simulink model "CC3"  (Simulink 7.5)
settings: Solver=ode45  StartTime=0.0  StopTime=2  RelTol=1e-3
(part 1 of 2)
settings Model: Creator=Fer  LastModifiedBy=Fer

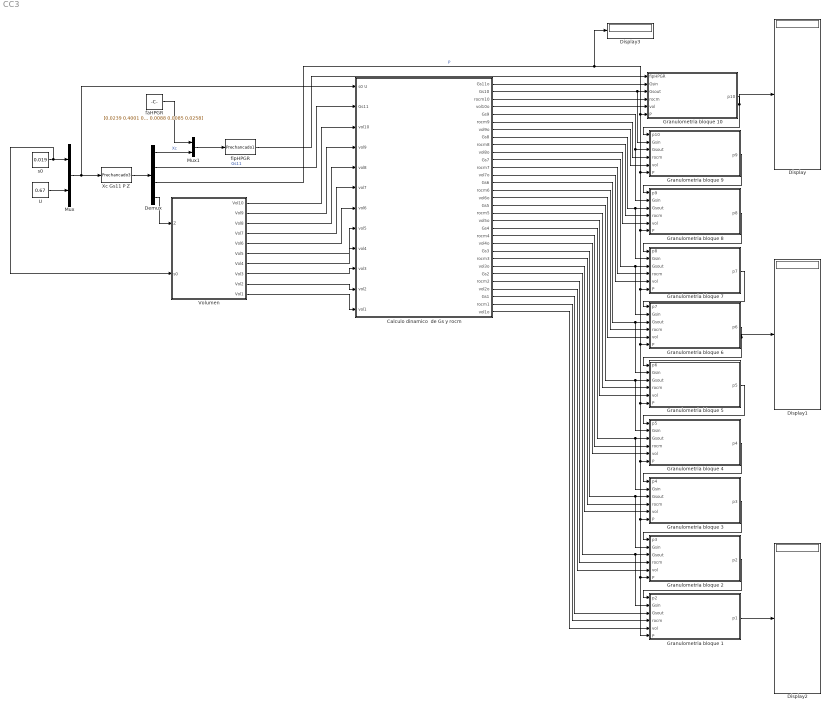
== system CC3 ==
  Calculo dinamico  de Gs y rocm : Subsystem
  Demux : Demux
  Display{,1..3} (4 alike) : Display
  Granulometria bloque 1 : Subsystem
  Granulometria bloque 10 : Subsystem
  Granulometria bloque 2 : Subsystem
  Granulometria bloque 3 : Subsystem
  Granulometria bloque 4 : Subsystem
  Granulometria bloque 5 : Subsystem
  Granulometria bloque 6 : Subsystem
  Granulometria bloque 7 : Subsystem
  Granulometria bloque 8 : Subsystem
  Granulometria bloque 9 : Subsystem
  Mux : Mux  Inputs=2
  Mux1 : Mux  Inputs=2
  U : Constant  Value=0.67  OutDataType=fixdt(1, 16)  OutScaling=2^0
  Volumen : Subsystem
  Xc Gs11 P Z : MATLABFcn  MATLABFcn=Prechancado3
  faHPGR : Constant  Value=[0.0239 0.4001 0.2089 0.1090 0.0549 0.0441 0.0542 0.0374 0.0159 0.0085 0.0088 0.0085 0.0258]  OutDataType=fixdt(1, 16)  OutScaling=2^0
  fipHPGR : MATLABFcn  MATLABFcn=Prechancado1
  s0 : Constant  Value=0.019  OutDataType=fixdt(1, 16)  OutScaling=2^0
  wires:
  s0/1 -> Mux/1, Volumen/2(s0)
  U/1 -> Mux/2
  Mux/1 -> Xc Gs11 P Z/1, Calculo dinamico  de Gs y rocm/1(s0 U)
  Xc Gs11 P Z/1 -> Demux/1
  faHPGR/1 -> Mux1/1
  Demux/1 -> Mux1/2  "Xc"
  Mux1/1 -> fipHPGR/1
  Demux/2 -> Calculo dinamico  de Gs y rocm/2(Gs11)  "Gs11"
  Volumen/1(Vol10) -> Calculo dinamico  de Gs y rocm/3(vol10)
  Volumen/2(Vol9) -> Calculo dinamico  de Gs y rocm/4(vol9)
  Volumen/3(Vol8) -> Calculo dinamico  de Gs y rocm/5(vol8)
  Volumen/4(Vol7) -> Calculo dinamico  de Gs y rocm/6(vol7)
  Volumen/5(Vol6) -> Calculo dinamico  de Gs y rocm/7(vol6)
  Volumen/6(Vol5) -> Calculo dinamico  de Gs y rocm/8(vol5)
  Volumen/7(Vol4) -> Calculo dinamico  de Gs y rocm/9(vol4)
  Volumen/8(Vol3) -> Calculo dinamico  de Gs y rocm/10(vol3)
  Volumen/9(Vol2) -> Calculo dinamico  de Gs y rocm/11(vol2)
  Volumen/10(Vol1) -> Calculo dinamico  de Gs y rocm/12(vol1)
  fipHPGR/1 -> Granulometria bloque 10/1(fipHPGR)
  Calculo dinamico  de Gs y rocm/1(Gs11o) -> Granulometria bloque 10/2(Gsin)
  Calculo dinamico  de Gs y rocm/2(Gs10) -> Granulometria bloque 10/3(Gsout), Granulometria bloque 9/2(Gsin)
  Calculo dinamico  de Gs y rocm/3(rocm10) -> Granulometria bloque 10/4(rocm)
  Calculo dinamico  de Gs y rocm/4(vol10o) -> Granulometria bloque 10/5(vol)
  Demux/4 -> Volumen/1(Z)
  Demux/3 -> Granulometria bloque 10/6(P), Granulometria bloque 9/6(P), Granulometria bloque 8/6(P), Granulometria bloque 7/6(P), Granulometria bloque 6/6(P), Granulometria bloque 5/6(P), Granulometria bloque 4/6(P), Granulometria bloque 3/6(P), Granulometria bloque 2/6(P), Granulometria bloque 1/6(P), Display3/1  "P"
  Granulometria bloque 10/1(p10) -> Granulometria bloque 9/1(p10), Display/1
  Calculo dinamico  de Gs y rocm/5(Gs9) -> Granulometria bloque 9/3(Gsout), Granulometria bloque 8/2(Gsin)
  Calculo dinamico  de Gs y rocm/6(rocm9) -> Granulometria bloque 9/4(rocm)
  Calculo dinamico  de Gs y rocm/7(vol9o) -> Granulometria bloque 9/5(vol)
  Granulometria bloque 9/1(p9) -> Granulometria bloque 8/1(p9)
  Calculo dinamico  de Gs y rocm/8(Gs8) -> Granulometria bloque 8/3(Gsout), Granulometria bloque 7/2(Gsin)
  Calculo dinamico  de Gs y rocm/9(rocm8) -> Granulometria bloque 8/4(rocm)
  Calculo dinamico  de Gs y rocm/10(vol8o) -> Granulometria bloque 8/5(vol)
  Granulometria bloque 8/1(p8) -> Granulometria bloque 7/1(p8)
  Calculo dinamico  de Gs y rocm/11(Gs7) -> Granulometria bloque 7/3(Gsout), Granulometria bloque 6/2(Gsin)
  Calculo dinamico  de Gs y rocm/12(rocm7) -> Granulometria bloque 7/4(rocm)
  Calculo dinamico  de Gs y rocm/13(vol7o) -> Granulometria bloque 7/5(vol)
  Granulometria bloque 7/1(p7) -> Granulometria bloque 6/1(p7)
  Calculo dinamico  de Gs y rocm/14(Gs6) -> Granulometria bloque 6/3(Gsout), Granulometria bloque 5/2(Gsin)
  Calculo dinamico  de Gs y rocm/15(rocm6) -> Granulometria bloque 6/4(rocm)
  Calculo dinamico  de Gs y rocm/16(vol6o) -> Granulometria bloque 6/5(vol)
  Granulometria bloque 6/1(p6) -> Granulometria bloque 5/1(p6), Display1/1
  Calculo dinamico  de Gs y rocm/17(Gs5) -> Granulometria bloque 5/3(Gsout), Granulometria bloque 4/2(Gsin)
  Calculo dinamico  de Gs y rocm/18(rocm5) -> Granulometria bloque 5/4(rocm)
  Calculo dinamico  de Gs y rocm/19(vol5o) -> Granulometria bloque 5/5(vol)
  Granulometria bloque 5/1(p5) -> Granulometria bloque 4/1(p5)
  Calculo dinamico  de Gs y rocm/20(Gs4) -> Granulometria bloque 4/3(Gsout), Granulometria bloque 3/2(Gsin)
  Calculo dinamico  de Gs y rocm/21(rocm4) -> Granulometria bloque 4/4(rocm)
  Calculo dinamico  de Gs y rocm/22(vol4o) -> Granulometria bloque 4/5(vol)
  Granulometria bloque 4/1(p4) -> Granulometria bloque 3/1(p4)
  Calculo dinamico  de Gs y rocm/23(Gs3) -> Granulometria bloque 3/3(Gsout), Granulometria bloque 2/2(Gsin)
  Calculo dinamico  de Gs y rocm/24(rocm3) -> Granulometria bloque 3/4(rocm)
  Calculo dinamico  de Gs y rocm/25(vol3o) -> Granulometria bloque 3/5(vol)
  Granulometria bloque 3/1(p3) -> Granulometria bloque 2/1(p3)
  Calculo dinamico  de Gs y rocm/26(Gs2) -> Granulometria bloque 2/3(Gsout), Granulometria bloque 1/2(Gsin)
  Calculo dinamico  de Gs y rocm/27(rocm2) -> Granulometria bloque 2/4(rocm)
  Calculo dinamico  de Gs y rocm/28(vol2o) -> Granulometria bloque 2/5(vol)
  Granulometria bloque 2/1(p2) -> Granulometria bloque 1/1(p2)
  Calculo dinamico  de Gs y rocm/29(Gs1) -> Granulometria bloque 1/3(Gsout)
  Calculo dinamico  de Gs y rocm/30(rocm1) -> Granulometria bloque 1/4(rocm)
  Calculo dinamico  de Gs y rocm/31(vol1o) -> Granulometria bloque 1/5(vol)
  Granulometria bloque 1/1(p1) -> Display2/1

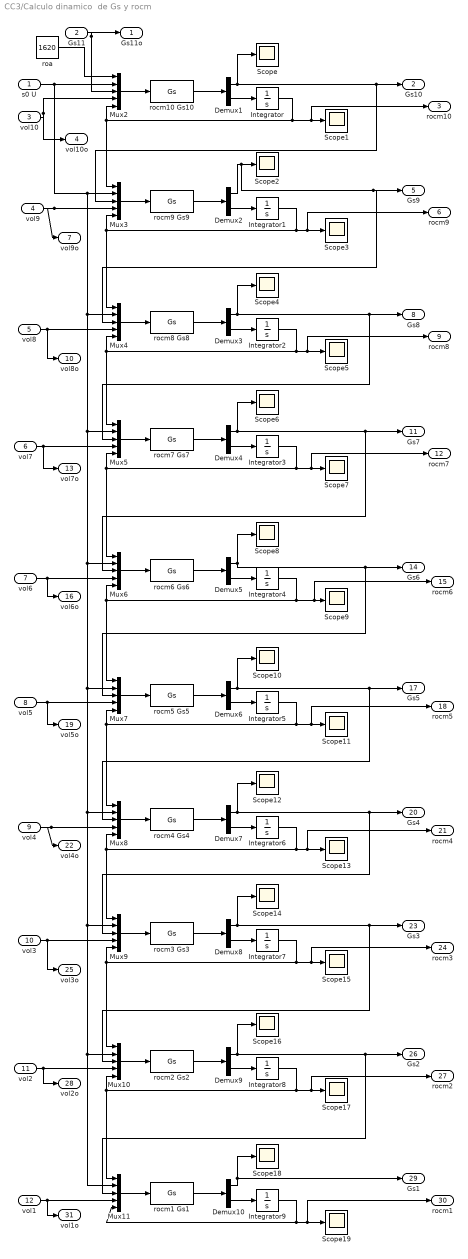
== system CC3/Calculo dinamico  de Gs y rocm ==
  s0 U : Inport
  Gs11 : Inport  Port=2
  vol10 : Inport  Port=3
  vol9 : Inport  Port=4
  vol8 : Inport  Port=5
  vol7 : Inport  Port=6
  vol6 : Inport  Port=7
  vol5 : Inport  Port=8
  vol4 : Inport  Port=9
  vol3 : Inport  Port=10
  vol2 : Inport  Port=11
  vol1 : Inport  Port=12
  Demux{1..10} (10 alike) : Demux  Outputs=2
  Integrator{,1..9} (10 alike) : Integrator  InitialCondition=1600
  Mux{2..11} (10 alike) : Mux  Inputs=5
  Scope{,1..19} (20 alike) : Scope
      Scope10 settings: SaveName=ScopeData10
      Scope11 settings: TimeRange=10  SaveName=ScopeData11
      Scope12 settings: SaveName=ScopeData12
      Scope13 settings: TimeRange=10  SaveName=ScopeData13
      Scope14 settings: SaveName=ScopeData14
      Scope15 settings: TimeRange=10  SaveName=ScopeData15
      Scope16 settings: SaveName=ScopeData16
      Scope17 settings: TimeRange=10  SaveName=ScopeData17
      Scope18 settings: SaveName=ScopeData18
      Scope19 settings: TimeRange=10  SaveName=ScopeData19
      Scope2 settings: SaveName=ScopeData2
      Scope3 settings: SaveName=ScopeData3
      Scope4 settings: SaveName=ScopeData4
      Scope5 settings: SaveName=ScopeData5
      Scope6 settings: SaveName=ScopeData6
      Scope7 settings: SaveName=ScopeData7
      Scope8 settings: SaveName=ScopeData8
      Scope9 settings: SaveName=ScopeData9
  roa : Constant  Value=1620  OutDataType=fixdt(1, 16)  OutScaling=2^0
  rocm1 Gs1 : MATLABFcn  MATLABFcn=Gs
  rocm10 Gs10 : MATLABFcn  MATLABFcn=Gs
  rocm2 Gs2 : MATLABFcn  MATLABFcn=Gs
  rocm3 Gs3 : MATLABFcn  MATLABFcn=Gs
  rocm4 Gs4 : MATLABFcn  MATLABFcn=Gs
  rocm5 Gs5 : MATLABFcn  MATLABFcn=Gs
  rocm6 Gs6 : MATLABFcn  MATLABFcn=Gs
  rocm7 Gs7 : MATLABFcn  MATLABFcn=Gs
  rocm8 Gs8 : MATLABFcn  MATLABFcn=Gs
  rocm9 Gs9 : MATLABFcn  MATLABFcn=Gs
  Gs11o : Outport  OutDataType=fixdt(1, 16)  OutScaling=2^0
  Gs10 : Outport  Port=2  OutDataType=fixdt(1, 16)  OutScaling=2^0
  rocm10 : Outport  Port=3  OutDataType=fixdt(1, 16)  OutScaling=2^0
  vol10o : Outport  Port=4  OutDataType=fixdt(1, 16)  OutScaling=2^0
  Gs9 : Outport  Port=5  OutDataType=fixdt(1, 16)  OutScaling=2^0
  rocm9 : Outport  Port=6  OutDataType=fixdt(1, 16)  OutScaling=2^0
  vol9o : Outport  Port=7  OutDataType=fixdt(1, 16)  OutScaling=2^0
  Gs8 : Outport  Port=8  OutDataType=fixdt(1, 16)  OutScaling=2^0
  rocm8 : Outport  Port=9  OutDataType=fixdt(1, 16)  OutScaling=2^0
  vol8o : Outport  Port=10  OutDataType=fixdt(1, 16)  OutScaling=2^0
  Gs7 : Outport  Port=11  OutDataType=fixdt(1, 16)  OutScaling=2^0
  rocm7 : Outport  Port=12  OutDataType=fixdt(1, 16)  OutScaling=2^0
  vol7o : Outport  Port=13  OutDataType=fixdt(1, 16)  OutScaling=2^0
  Gs6 : Outport  Port=14  OutDataType=fixdt(1, 16)  OutScaling=2^0
  rocm6 : Outport  Port=15  OutDataType=fixdt(1, 16)  OutScaling=2^0
  vol6o : Outport  Port=16  OutDataType=fixdt(1, 16)  OutScaling=2^0
  Gs5 : Outport  Port=17  OutDataType=fixdt(1, 16)  OutScaling=2^0
  rocm5 : Outport  Port=18  OutDataType=fixdt(1, 16)  OutScaling=2^0
  vol5o : Outport  Port=19  OutDataType=fixdt(1, 16)  OutScaling=2^0
  Gs4 : Outport  Port=20  OutDataType=fixdt(1, 16)  OutScaling=2^0
  rocm4 : Outport  Port=21  OutDataType=fixdt(1, 16)  OutScaling=2^0
  vol4o : Outport  Port=22  OutDataType=fixdt(1, 16)  OutScaling=2^0
  Gs3 : Outport  Port=23  OutDataType=fixdt(1, 16)  OutScaling=2^0
  rocm3 : Outport  Port=24  OutDataType=fixdt(1, 16)  OutScaling=2^0
  vol3o : Outport  Port=25  OutDataType=fixdt(1, 16)  OutScaling=2^0
  Gs2 : Outport  Port=26  OutDataType=fixdt(1, 16)  OutScaling=2^0
  rocm2 : Outport  Port=27  OutDataType=fixdt(1, 16)  OutScaling=2^0
  vol2o : Outport  Port=28  OutDataType=fixdt(1, 16)  OutScaling=2^0
  Gs1 : Outport  Port=29  OutDataType=fixdt(1, 16)  OutScaling=2^0
  rocm1 : Outport  Port=30  OutDataType=fixdt(1, 16)  OutScaling=2^0
  vol1o : Outport  Port=31  OutDataType=fixdt(1, 16)  OutScaling=2^0
  wires:
  Mux2/1 -> rocm10 Gs10/1
  rocm10 Gs10/1 -> Demux1/1
  Demux1/1 -> Scope/1, Mux3/3, Gs10/1
  Demux1/2 -> Integrator/1
  Integrator/1 -> Mux2/5, Mux3/1, Scope1/1, rocm10/1
  roa/1 -> Mux2/1
  Mux3/1 -> rocm9 Gs9/1
  rocm9 Gs9/1 -> Demux2/1
  Demux2/1 -> Scope2/1, Mux4/3, Gs9/1
  Demux2/2 -> Integrator1/1
  Integrator1/1 -> Mux3/5, Mux4/1, Scope3/1, rocm9/1
  Mux4/1 -> rocm8 Gs8/1
  rocm8 Gs8/1 -> Demux3/1
  Demux3/1 -> Scope4/1, Mux5/3, Gs8/1
  Demux3/2 -> Integrator2/1
  Integrator2/1 -> Mux4/5, Mux5/1, Scope5/1, rocm8/1
  rocm7 Gs7/1 -> Demux4/1
  Demux4/1 -> Scope6/1, Mux6/3, Gs7/1
  Demux4/2 -> Integrator3/1
  Integrator3/1 -> Mux5/5, Mux6/1, Scope7/1, rocm7/1
  Mux5/1 -> rocm7 Gs7/1
  Mux6/1 -> rocm6 Gs6/1
  rocm6 Gs6/1 -> Demux5/1
  Demux5/1 -> Scope8/1, Mux7/3, Gs6/1
  Demux5/2 -> Integrator4/1
  Integrator4/1 -> Mux6/5, Mux7/1, Scope9/1, rocm6/1
  Mux7/1 -> rocm5 Gs5/1
  rocm5 Gs5/1 -> Demux6/1
  Demux6/1 -> Scope10/1, Mux8/3, Gs5/1
  Demux6/2 -> Integrator5/1
  Integrator5/1 -> Mux7/5, Mux8/1, Scope11/1, rocm5/1
  rocm4 Gs4/1 -> Demux7/1
  Demux7/1 -> Scope12/1, Mux9/3, Gs4/1
  Demux7/2 -> Integrator6/1
  Integrator6/1 -> Mux8/5, Mux9/1, Scope13/1, rocm4/1
  Mux8/1 -> rocm4 Gs4/1
  rocm3 Gs3/1 -> Demux8/1
  Demux8/1 -> Scope14/1, Mux10/3, Gs3/1
  Demux8/2 -> Integrator7/1
  Integrator7/1 -> Mux9/5, Mux10/1, Scope15/1, rocm3/1
  Mux9/1 -> rocm3 Gs3/1
  Demux9/2 -> Integrator8/1
  Integrator8/1 -> Mux10/5, Mux11/1, Scope17/1, rocm2/1
  rocm2 Gs2/1 -> Demux9/1
  Mux10/1 -> rocm2 Gs2/1
  Demux9/1 -> Scope16/1, Gs2/1, Mux11/3
  Mux11/1 -> rocm1 Gs1/1
  rocm1 Gs1/1 -> Demux10/1
  Demux10/2 -> Integrator9/1
  Integrator9/1 -> Mux11/5, Scope19/1, rocm1/1
  Demux10/1 -> Scope18/1, Gs1/1
  s0 U/1 -> Mux2/2, Mux3/2, Mux4/2, Mux5/2, Mux6/2, Mux7/2, Mux8/2, Mux9/2, Mux10/2, Mux11/2
  Gs11/1 -> Mux2/3, Gs11o/1
  vol10/1 -> Mux2/4, vol10o/1
  vol9/1 -> Mux3/4, vol9o/1
  vol8/1 -> Mux4/4, vol8o/1
  vol7/1 -> Mux5/4, vol7o/1
  vol6/1 -> Mux6/4, vol6o/1
  vol5/1 -> Mux7/4, vol5o/1
  vol4/1 -> Mux8/4, vol4o/1
  vol3/1 -> Mux9/4, vol3o/1
  vol2/1 -> Mux10/4, vol2o/1
  vol1/1 -> Mux11/4, vol1o/1

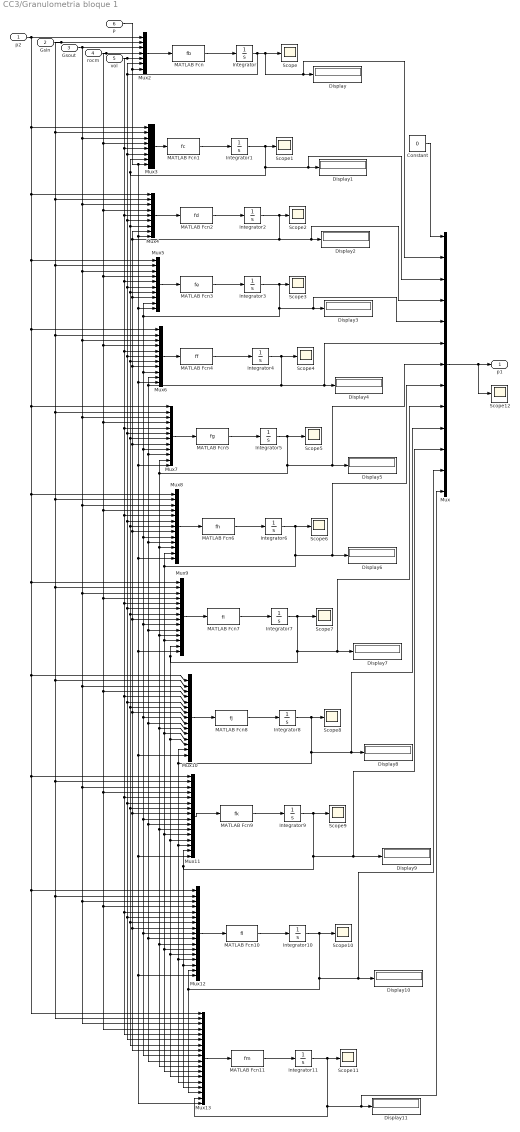
== system CC3/Granulometria bloque 1 ==
  p2 : Inport
  Gsin : Inport  Port=2
  Gsout : Inport  Port=3
  rocm : Inport  Port=4
  vol : Inport  Port=5
  P : Inport  Port=6
  Constant : Constant  Value=0  OutDataType=fixdt(1, 16)  OutScaling=2^0
  Display{,1..11} (12 alike) : Display
  Integrator{,1..11} (12 alike) : Integrator  InitialCondition=0.003
  MATLAB Fcn : MATLABFcn  MATLABFcn=fb
  MATLAB Fcn1 : MATLABFcn  MATLABFcn=fc
  MATLAB Fcn10 : MATLABFcn  MATLABFcn=fl
  MATLAB Fcn11 : MATLABFcn  MATLABFcn=fm
  MATLAB Fcn2 : MATLABFcn  MATLABFcn=fd
  MATLAB Fcn3 : MATLABFcn  MATLABFcn=fe
  MATLAB Fcn4 : MATLABFcn  MATLABFcn=ff
  MATLAB Fcn5 : MATLABFcn  MATLABFcn=fg
  MATLAB Fcn6 : MATLABFcn  MATLABFcn=fh
  MATLAB Fcn7 : MATLABFcn  MATLABFcn=fi
  MATLAB Fcn8 : MATLABFcn  MATLABFcn=fj
  MATLAB Fcn9 : MATLABFcn  MATLABFcn=fk
  Mux : Mux  Inputs=13
  Mux10 : Mux  Inputs=15
  Mux11 : Mux  Inputs=16
  Mux12 : Mux  Inputs=17
  Mux13 : Mux  Inputs=18
  Mux2 : Mux  Inputs=7
  Mux3 : Mux  Inputs=8
  Mux4 : Mux  Inputs=9
  Mux5 : Mux  Inputs=10
  Mux6 : Mux  Inputs=11
  Mux7 : Mux  Inputs=12
  Mux8 : Mux  Inputs=13
  Mux9 : Mux  Inputs=14
  Scope{,1..12} (13 alike) : Scope
      Scope settings: SaveName=ScopeData2
      Scope1 settings: SaveName=ScopeData20
      Scope10 settings: SaveName=ScopeData29
      Scope11 settings: SaveName=ScopeData30
      Scope12 settings: SaveName=ScopeData39
      Scope2 settings: SaveName=ScopeData21
      Scope3 settings: SaveName=ScopeData22
      Scope4 settings: SaveName=ScopeData23
      Scope5 settings: SaveName=ScopeData24
      Scope6 settings: SaveName=ScopeData25
      Scope7 settings: SaveName=ScopeData26
      Scope8 settings: SaveName=ScopeData27
      Scope9 settings: SaveName=ScopeData28
  p1 : Outport  OutDataType=fixdt(1, 16)  OutScaling=2^0
  wires:
  Mux2/1 -> MATLAB Fcn/1
  MATLAB Fcn/1 -> Integrator/1
  Integrator/1 -> Mux2/6, Mux3/6, Mux4/6, Mux5/6, Mux6/6, Mux7/6, Mux8/6, Mux9/6, Mux10/6, Mux11/6, Mux12/6, Mux13/6, Scope/1, Display/1, Mux/2
  p2/1 -> Mux2/1, Mux3/1, Mux4/1, Mux5/1, Mux6/1, Mux7/1, Mux8/1, Mux9/1, Mux10/1, Mux11/1, Mux12/1, Mux13/1
  Gsin/1 -> Mux2/2, Mux3/2, Mux4/2, Mux5/2, Mux6/2, Mux7/2, Mux8/2, Mux9/2, Mux10/2, Mux11/2, Mux12/2, Mux13/2
  Gsout/1 -> Mux2/3, Mux3/3, Mux4/3, Mux5/3, Mux6/3, Mux7/3, Mux8/3, Mux9/3, Mux10/3, Mux11/3, Mux12/3, Mux13/3
  rocm/1 -> Mux2/4, Mux3/4, Mux4/4, Mux5/4, Mux6/4, Mux7/4, Mux8/4, Mux9/4, Mux10/4, Mux11/4, Mux12/4, Mux13/4
  vol/1 -> Mux2/5, Mux3/5, Mux4/5, Mux5/5, Mux6/5, Mux7/5, Mux8/5, Mux9/5, Mux10/5, Mux11/5, Mux12/5, Mux13/5
  Mux3/1 -> MATLAB Fcn1/1
  MATLAB Fcn1/1 -> Integrator1/1
  Integrator1/1 -> Scope1/1, Mux3/7, Mux4/7, Mux5/7, Mux6/7, Mux7/7, Mux8/7, Mux9/7, Mux10/7, Mux11/7, Mux12/7, Mux13/7, Display1/1, Mux/3
  Mux4/1 -> MATLAB Fcn2/1
  MATLAB Fcn2/1 -> Integrator2/1
  Integrator2/1 -> Scope2/1, Mux4/8, Mux5/8, Mux6/8, Mux7/8, Mux8/8, Mux9/8, Mux10/8, Mux11/8, Mux12/8, Mux13/8, Display2/1, Mux/4
  MATLAB Fcn3/1 -> Integrator3/1
  Integrator3/1 -> Scope3/1, Mux5/9, Mux6/9, Mux7/9, Mux8/9, Mux9/9, Mux10/9, Mux11/9, Mux12/9, Mux13/9, Display3/1, Mux/5
  Mux5/1 -> MATLAB Fcn3/1
  Mux6/1 -> MATLAB Fcn4/1
  MATLAB Fcn4/1 -> Integrator4/1
  Integrator4/1 -> Scope4/1, Mux6/10, Mux7/10, Mux8/10, Mux9/10, Mux10/10, Mux11/10, Mux12/10, Mux13/10, Display4/1, Mux/6
  Mux7/1 -> MATLAB Fcn5/1
  MATLAB Fcn5/1 -> Integrator5/1
  Integrator5/1 -> Scope5/1, Mux7/11, Mux8/11, Mux9/11, Mux10/11, Mux11/11, Mux12/11, Mux13/11, Display5/1, Mux/7
  Mux8/1 -> MATLAB Fcn6/1
  MATLAB Fcn6/1 -> Integrator6/1
  Integrator6/1 -> Scope6/1, Mux8/12, Mux9/12, Mux10/12, Mux11/12, Mux12/12, Mux13/12, Display6/1, Mux/8
  Mux9/1 -> MATLAB Fcn7/1
  MATLAB Fcn7/1 -> Integrator7/1
  Integrator7/1 -> Scope7/1, Mux9/13, Mux10/13, Mux11/13, Mux12/13, Mux13/13, Display7/1, Mux/9
  Mux10/1 -> MATLAB Fcn8/1
  MATLAB Fcn8/1 -> Integrator8/1
  Integrator8/1 -> Scope8/1, Mux10/14, Mux11/14, Mux12/14, Mux13/14, Display8/1, Mux/10
  Mux11/1 -> MATLAB Fcn9/1
  MATLAB Fcn9/1 -> Integrator9/1
  Integrator9/1 -> Scope9/1, Mux11/15, Mux12/15, Mux13/15, Display9/1, Mux/11
  Mux12/1 -> MATLAB Fcn10/1
  MATLAB Fcn10/1 -> Integrator10/1
  Integrator10/1 -> Scope10/1, Mux12/16, Mux13/16, Display10/1, Mux/12
  Mux13/1 -> MATLAB Fcn11/1
  MATLAB Fcn11/1 -> Integrator11/1
  Integrator11/1 -> Scope11/1, Mux13/17, Display11/1, Mux/13
  Constant/1 -> Mux/1
  Mux/1 -> p1/1, Scope12/1
  P/1 -> Mux2/7, Mux3/8, Mux4/9, Mux5/10, Mux6/11, Mux7/12, Mux8/13, Mux9/14, Mux10/15, Mux11/16, Mux12/17, Mux13/18

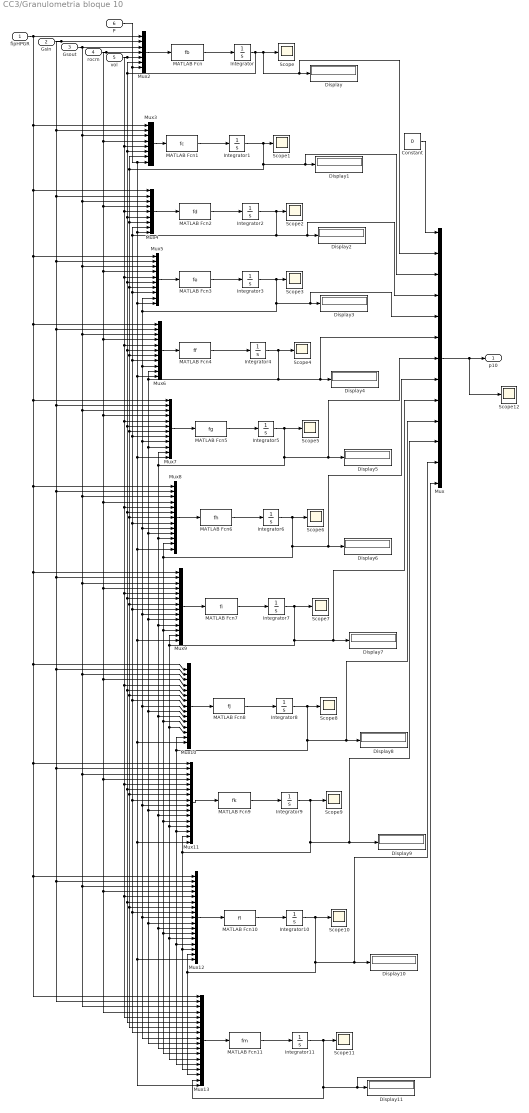
== system CC3/Granulometria bloque 10 ==
  fipHPGR : Inport
  Gsin : Inport  Port=2
  Gsout : Inport  Port=3
  rocm : Inport  Port=4
  vol : Inport  Port=5
  P : Inport  Port=6
  Constant : Constant  Value=0  OutDataType=fixdt(1, 16)  OutScaling=2^0
  Display{,1..11} (12 alike) : Display
  Integrator{,1..11} (12 alike) : Integrator  InitialCondition=0.003
  MATLAB Fcn : MATLABFcn  MATLABFcn=fb
  MATLAB Fcn1 : MATLABFcn  MATLABFcn=fc
  MATLAB Fcn10 : MATLABFcn  MATLABFcn=fl
  MATLAB Fcn11 : MATLABFcn  MATLABFcn=fm
  MATLAB Fcn2 : MATLABFcn  MATLABFcn=fd
  MATLAB Fcn3 : MATLABFcn  MATLABFcn=fe
  MATLAB Fcn4 : MATLABFcn  MATLABFcn=ff
  MATLAB Fcn5 : MATLABFcn  MATLABFcn=fg
  MATLAB Fcn6 : MATLABFcn  MATLABFcn=fh
  MATLAB Fcn7 : MATLABFcn  MATLABFcn=fi
  MATLAB Fcn8 : MATLABFcn  MATLABFcn=fj
  MATLAB Fcn9 : MATLABFcn  MATLABFcn=fk
  Mux : Mux  Inputs=13
  Mux10 : Mux  Inputs=15
  Mux11 : Mux  Inputs=16
  Mux12 : Mux  Inputs=17
  Mux13 : Mux  Inputs=18
  Mux2 : Mux  Inputs=7
  Mux3 : Mux  Inputs=8
  Mux4 : Mux  Inputs=9
  Mux5 : Mux  Inputs=10
  Mux6 : Mux  Inputs=11
  Mux7 : Mux  Inputs=12
  Mux8 : Mux  Inputs=13
  Mux9 : Mux  Inputs=14
  Scope{,1..12} (13 alike) : Scope
      Scope settings: SaveName=ScopeData2
      Scope1 settings: SaveName=ScopeData20
      Scope10 settings: SaveName=ScopeData29
      Scope11 settings: SaveName=ScopeData30
      Scope12 settings: SaveName=ScopeData2
      Scope2 settings: SaveName=ScopeData21
      Scope3 settings: SaveName=ScopeData22
      Scope4 settings: SaveName=ScopeData23
      Scope5 settings: SaveName=ScopeData24
      Scope6 settings: SaveName=ScopeData25
      Scope7 settings: SaveName=ScopeData26
      Scope8 settings: SaveName=ScopeData27
      Scope9 settings: SaveName=ScopeData28
  p10 : Outport  OutDataType=fixdt(1, 16)  OutScaling=2^0
  wires:
  Mux2/1 -> MATLAB Fcn/1
  MATLAB Fcn/1 -> Integrator/1
  Integrator/1 -> Mux2/6, Mux3/6, Mux4/6, Mux5/6, Mux6/6, Mux7/6, Mux8/6, Mux9/6, Mux10/6, Mux11/6, Mux12/6, Mux13/6, Scope/1, Display/1, Mux/2
  fipHPGR/1 -> Mux2/1, Mux3/1, Mux4/1, Mux5/1, Mux6/1, Mux7/1, Mux8/1, Mux9/1, Mux10/1, Mux11/1, Mux12/1, Mux13/1
  Gsin/1 -> Mux2/2, Mux3/2, Mux4/2, Mux5/2, Mux6/2, Mux7/2, Mux8/2, Mux9/2, Mux10/2, Mux11/2, Mux12/2, Mux13/2
  Gsout/1 -> Mux2/3, Mux3/3, Mux4/3, Mux5/3, Mux6/3, Mux7/3, Mux8/3, Mux9/3, Mux10/3, Mux11/3, Mux12/3, Mux13/3
  rocm/1 -> Mux2/4, Mux3/4, Mux4/4, Mux5/4, Mux6/4, Mux7/4, Mux8/4, Mux9/4, Mux10/4, Mux11/4, Mux12/4, Mux13/4
  vol/1 -> Mux2/5, Mux3/5, Mux4/5, Mux5/5, Mux6/5, Mux7/5, Mux8/5, Mux9/5, Mux10/5, Mux11/5, Mux12/5, Mux13/5
  Mux3/1 -> MATLAB Fcn1/1
  MATLAB Fcn1/1 -> Integrator1/1
  Integrator1/1 -> Scope1/1, Mux3/7, Mux4/7, Mux5/7, Mux6/7, Mux7/7, Mux8/7, Mux9/7, Mux10/7, Mux11/7, Mux12/7, Mux13/7, Display1/1, Mux/3
  Mux4/1 -> MATLAB Fcn2/1
  MATLAB Fcn2/1 -> Integrator2/1
  Integrator2/1 -> Scope2/1, Mux4/8, Mux5/8, Mux6/8, Mux7/8, Mux8/8, Mux9/8, Mux10/8, Mux11/8, Mux12/8, Mux13/8, Display2/1, Mux/4
  MATLAB Fcn3/1 -> Integrator3/1
  Integrator3/1 -> Scope3/1, Mux5/9, Mux6/9, Mux7/9, Mux8/9, Mux9/9, Mux10/9, Mux11/9, Mux12/9, Mux13/9, Display3/1, Mux/5
  Mux5/1 -> MATLAB Fcn3/1
  Mux6/1 -> MATLAB Fcn4/1
  MATLAB Fcn4/1 -> Integrator4/1
  Integrator4/1 -> Scope4/1, Mux6/10, Mux7/10, Mux8/10, Mux9/10, Mux10/10, Mux11/10, Mux12/10, Mux13/10, Display4/1, Mux/6
  Mux7/1 -> MATLAB Fcn5/1
  MATLAB Fcn5/1 -> Integrator5/1
  Integrator5/1 -> Scope5/1, Mux7/11, Mux8/11, Mux9/11, Mux10/11, Mux11/11, Mux12/11, Mux13/11, Display5/1, Mux/7
  Mux8/1 -> MATLAB Fcn6/1
  MATLAB Fcn6/1 -> Integrator6/1
  Integrator6/1 -> Scope6/1, Mux8/12, Mux9/12, Mux10/12, Mux11/12, Mux12/12, Mux13/12, Display6/1, Mux/8
  Mux9/1 -> MATLAB Fcn7/1
  MATLAB Fcn7/1 -> Integrator7/1
  Integrator7/1 -> Scope7/1, Mux9/13, Mux10/13, Mux11/13, Mux12/13, Mux13/13, Display7/1, Mux/9
  Mux10/1 -> MATLAB Fcn8/1
  MATLAB Fcn8/1 -> Integrator8/1
  Integrator8/1 -> Scope8/1, Mux10/14, Mux11/14, Mux12/14, Mux13/14, Display8/1, Mux/10
  Mux11/1 -> MATLAB Fcn9/1
  MATLAB Fcn9/1 -> Integrator9/1
  Integrator9/1 -> Scope9/1, Mux11/15, Mux12/15, Mux13/15, Display9/1, Mux/11
  Mux12/1 -> MATLAB Fcn10/1
  MATLAB Fcn10/1 -> Integrator10/1
  Integrator10/1 -> Scope10/1, Mux12/16, Mux13/16, Display10/1, Mux/12
  Mux13/1 -> MATLAB Fcn11/1
  MATLAB Fcn11/1 -> Integrator11/1
  Integrator11/1 -> Scope11/1, Mux13/17, Display11/1, Mux/13
  Constant/1 -> Mux/1
  Mux/1 -> p10/1, Scope12/1
  P/1 -> Mux2/7, Mux3/8, Mux4/9, Mux5/10, Mux6/11, Mux7/12, Mux8/13, Mux9/14, Mux10/15, Mux11/16, Mux12/17, Mux13/18

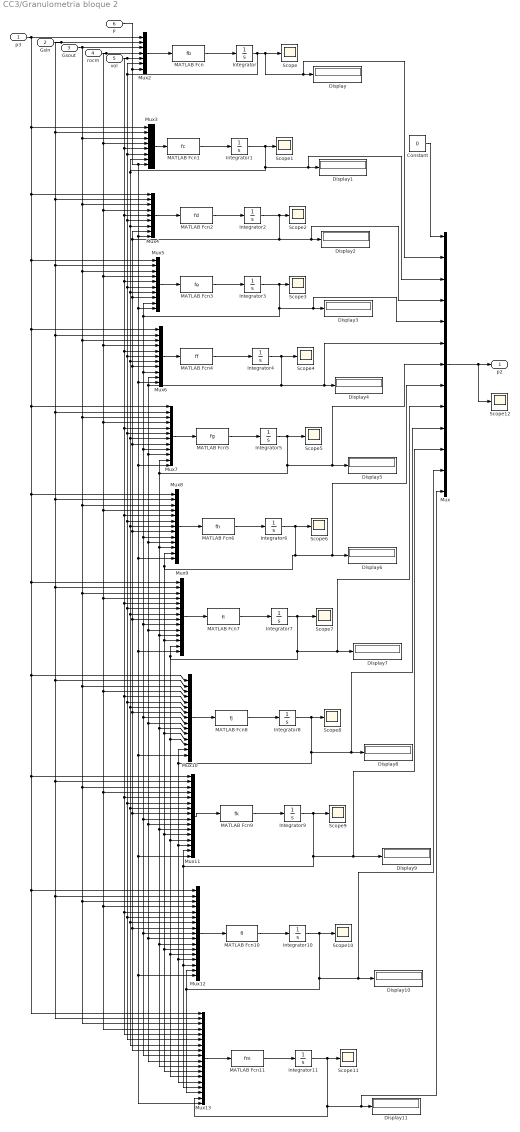
== system CC3/Granulometria bloque 2 ==
  p3 : Inport
  Gsin : Inport  Port=2
  Gsout : Inport  Port=3
  rocm : Inport  Port=4
  vol : Inport  Port=5
  P : Inport  Port=6
  Constant : Constant  Value=0  OutDataType=fixdt(1, 16)  OutScaling=2^0
  Display{,1..11} (12 alike) : Display
  Integrator{,1..11} (12 alike) : Integrator  InitialCondition=0.003
  MATLAB Fcn : MATLABFcn  MATLABFcn=fb
  MATLAB Fcn1 : MATLABFcn  MATLABFcn=fc
  MATLAB Fcn10 : MATLABFcn  MATLABFcn=fl
  MATLAB Fcn11 : MATLABFcn  MATLABFcn=fm
  MATLAB Fcn2 : MATLABFcn  MATLABFcn=fd
  MATLAB Fcn3 : MATLABFcn  MATLABFcn=fe
  MATLAB Fcn4 : MATLABFcn  MATLABFcn=ff
  MATLAB Fcn5 : MATLABFcn  MATLABFcn=fg
  MATLAB Fcn6 : MATLABFcn  MATLABFcn=fh
  MATLAB Fcn7 : MATLABFcn  MATLABFcn=fi
  MATLAB Fcn8 : MATLABFcn  MATLABFcn=fj
  MATLAB Fcn9 : MATLABFcn  MATLABFcn=fk
  Mux : Mux  Inputs=13
  Mux10 : Mux  Inputs=15
  Mux11 : Mux  Inputs=16
  Mux12 : Mux  Inputs=17
  Mux13 : Mux  Inputs=18
  Mux2 : Mux  Inputs=7
  Mux3 : Mux  Inputs=8
  Mux4 : Mux  Inputs=9
  Mux5 : Mux  Inputs=10
  Mux6 : Mux  Inputs=11
  Mux7 : Mux  Inputs=12
  Mux8 : Mux  Inputs=13
  Mux9 : Mux  Inputs=14
  Scope{,1..12} (13 alike) : Scope
      Scope settings: SaveName=ScopeData2
      Scope1 settings: SaveName=ScopeData20
      Scope10 settings: SaveName=ScopeData29
      Scope11 settings: SaveName=ScopeData30
      Scope12 settings: SaveName=ScopeData38
      Scope2 settings: SaveName=ScopeData21
      Scope3 settings: SaveName=ScopeData22
      Scope4 settings: SaveName=ScopeData23
      Scope5 settings: SaveName=ScopeData24
      Scope6 settings: SaveName=ScopeData25
      Scope7 settings: SaveName=ScopeData26
      Scope8 settings: SaveName=ScopeData27
      Scope9 settings: SaveName=ScopeData28
  p2 : Outport  OutDataType=fixdt(1, 16)  OutScaling=2^0
  wires:
  Mux2/1 -> MATLAB Fcn/1
  MATLAB Fcn/1 -> Integrator/1
  Integrator/1 -> Mux2/6, Mux3/6, Mux4/6, Mux5/6, Mux6/6, Mux7/6, Mux8/6, Mux9/6, Mux10/6, Mux11/6, Mux12/6, Mux13/6, Scope/1, Display/1, Mux/2
  p3/1 -> Mux2/1, Mux3/1, Mux4/1, Mux5/1, Mux6/1, Mux7/1, Mux8/1, Mux9/1, Mux10/1, Mux11/1, Mux12/1, Mux13/1
  Gsin/1 -> Mux2/2, Mux3/2, Mux4/2, Mux5/2, Mux6/2, Mux7/2, Mux8/2, Mux9/2, Mux10/2, Mux11/2, Mux12/2, Mux13/2
  Gsout/1 -> Mux2/3, Mux3/3, Mux4/3, Mux5/3, Mux6/3, Mux7/3, Mux8/3, Mux9/3, Mux10/3, Mux11/3, Mux12/3, Mux13/3
  rocm/1 -> Mux2/4, Mux3/4, Mux4/4, Mux5/4, Mux6/4, Mux7/4, Mux8/4, Mux9/4, Mux10/4, Mux11/4, Mux12/4, Mux13/4
  vol/1 -> Mux2/5, Mux3/5, Mux4/5, Mux5/5, Mux6/5, Mux7/5, Mux8/5, Mux9/5, Mux10/5, Mux11/5, Mux12/5, Mux13/5
  Mux3/1 -> MATLAB Fcn1/1
  MATLAB Fcn1/1 -> Integrator1/1
  Integrator1/1 -> Scope1/1, Mux3/7, Mux4/7, Mux5/7, Mux6/7, Mux7/7, Mux8/7, Mux9/7, Mux10/7, Mux11/7, Mux12/7, Mux13/7, Display1/1, Mux/3
  Mux4/1 -> MATLAB Fcn2/1
  MATLAB Fcn2/1 -> Integrator2/1
  Integrator2/1 -> Scope2/1, Mux4/8, Mux5/8, Mux6/8, Mux7/8, Mux8/8, Mux9/8, Mux10/8, Mux11/8, Mux12/8, Mux13/8, Display2/1, Mux/4
  MATLAB Fcn3/1 -> Integrator3/1
  Integrator3/1 -> Scope3/1, Mux5/9, Mux6/9, Mux7/9, Mux8/9, Mux9/9, Mux10/9, Mux11/9, Mux12/9, Mux13/9, Display3/1, Mux/5
  Mux5/1 -> MATLAB Fcn3/1
  Mux6/1 -> MATLAB Fcn4/1
  MATLAB Fcn4/1 -> Integrator4/1
  Integrator4/1 -> Scope4/1, Mux6/10, Mux7/10, Mux8/10, Mux9/10, Mux10/10, Mux11/10, Mux12/10, Mux13/10, Display4/1, Mux/6
  Mux7/1 -> MATLAB Fcn5/1
  MATLAB Fcn5/1 -> Integrator5/1
  Integrator5/1 -> Scope5/1, Mux7/11, Mux8/11, Mux9/11, Mux10/11, Mux11/11, Mux12/11, Mux13/11, Display5/1, Mux/7
  Mux8/1 -> MATLAB Fcn6/1
  MATLAB Fcn6/1 -> Integrator6/1
  Integrator6/1 -> Scope6/1, Mux8/12, Mux9/12, Mux10/12, Mux11/12, Mux12/12, Mux13/12, Display6/1, Mux/8
  Mux9/1 -> MATLAB Fcn7/1
  MATLAB Fcn7/1 -> Integrator7/1
  Integrator7/1 -> Scope7/1, Mux9/13, Mux10/13, Mux11/13, Mux12/13, Mux13/13, Display7/1, Mux/9
  Mux10/1 -> MATLAB Fcn8/1
  MATLAB Fcn8/1 -> Integrator8/1
  Integrator8/1 -> Scope8/1, Mux10/14, Mux11/14, Mux12/14, Mux13/14, Display8/1, Mux/10
  Mux11/1 -> MATLAB Fcn9/1
  MATLAB Fcn9/1 -> Integrator9/1
  Integrator9/1 -> Scope9/1, Mux11/15, Mux12/15, Mux13/15, Display9/1, Mux/11
  Mux12/1 -> MATLAB Fcn10/1
  MATLAB Fcn10/1 -> Integrator10/1
  Integrator10/1 -> Scope10/1, Mux12/16, Mux13/16, Display10/1, Mux/12
  Mux13/1 -> MATLAB Fcn11/1
  MATLAB Fcn11/1 -> Integrator11/1
  Integrator11/1 -> Scope11/1, Mux13/17, Display11/1, Mux/13
  Constant/1 -> Mux/1
  Mux/1 -> p2/1, Scope12/1
  P/1 -> Mux2/7, Mux3/8, Mux4/9, Mux5/10, Mux6/11, Mux7/12, Mux8/13, Mux9/14, Mux10/15, Mux11/16, Mux12/17, Mux13/18

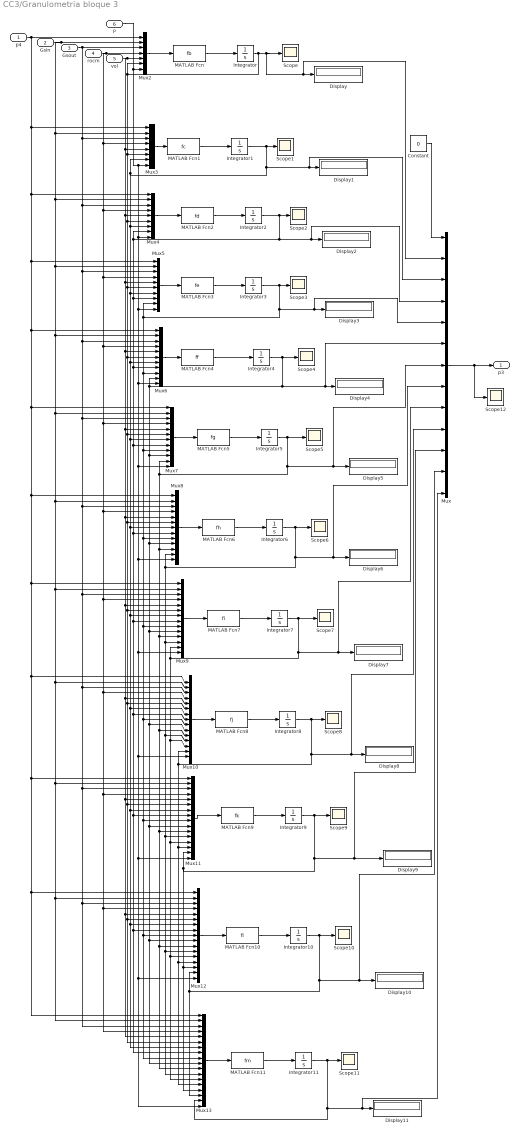
== system CC3/Granulometria bloque 3 ==
  p4 : Inport
  Gsin : Inport  Port=2
  Gsout : Inport  Port=3
  rocm : Inport  Port=4
  vol : Inport  Port=5
  P : Inport  Port=6
  Constant : Constant  Value=0  OutDataType=fixdt(1, 16)  OutScaling=2^0
  Display{,1..11} (12 alike) : Display
  Integrator{,1..11} (12 alike) : Integrator  InitialCondition=0.003
  MATLAB Fcn : MATLABFcn  MATLABFcn=fb
  MATLAB Fcn1 : MATLABFcn  MATLABFcn=fc
  MATLAB Fcn10 : MATLABFcn  MATLABFcn=fl
  MATLAB Fcn11 : MATLABFcn  MATLABFcn=fm
  MATLAB Fcn2 : MATLABFcn  MATLABFcn=fd
  MATLAB Fcn3 : MATLABFcn  MATLABFcn=fe
  MATLAB Fcn4 : MATLABFcn  MATLABFcn=ff
  MATLAB Fcn5 : MATLABFcn  MATLABFcn=fg
  MATLAB Fcn6 : MATLABFcn  MATLABFcn=fh
  MATLAB Fcn7 : MATLABFcn  MATLABFcn=fi
  MATLAB Fcn8 : MATLABFcn  MATLABFcn=fj
  MATLAB Fcn9 : MATLABFcn  MATLABFcn=fk
  Mux : Mux  Inputs=13
  Mux10 : Mux  Inputs=15
  Mux11 : Mux  Inputs=16
  Mux12 : Mux  Inputs=17
  Mux13 : Mux  Inputs=18
  Mux2 : Mux  Inputs=7
  Mux3 : Mux  Inputs=8
  Mux4 : Mux  Inputs=9
  Mux5 : Mux  Inputs=10
  Mux6 : Mux  Inputs=11
  Mux7 : Mux  Inputs=12
  Mux8 : Mux  Inputs=13
  Mux9 : Mux  Inputs=14
  Scope{,1..12} (13 alike) : Scope
      Scope settings: SaveName=ScopeData2
      Scope1 settings: SaveName=ScopeData20
      Scope10 settings: SaveName=ScopeData29
      Scope11 settings: SaveName=ScopeData30
      Scope12 settings: SaveName=ScopeData37
      Scope2 settings: SaveName=ScopeData21
      Scope3 settings: SaveName=ScopeData22
      Scope4 settings: SaveName=ScopeData23
      Scope5 settings: SaveName=ScopeData24
      Scope6 settings: SaveName=ScopeData25
      Scope7 settings: SaveName=ScopeData26
      Scope8 settings: SaveName=ScopeData27
      Scope9 settings: SaveName=ScopeData28
  p3 : Outport  OutDataType=fixdt(1, 16)  OutScaling=2^0
  wires:
  Mux2/1 -> MATLAB Fcn/1
  MATLAB Fcn/1 -> Integrator/1
  Integrator/1 -> Mux2/6, Mux3/6, Mux4/6, Mux5/6, Mux6/6, Mux7/6, Mux8/6, Mux9/6, Mux10/6, Mux11/6, Mux12/6, Mux13/6, Scope/1, Display/1, Mux/2
  p4/1 -> Mux2/1, Mux3/1, Mux4/1, Mux5/1, Mux6/1, Mux7/1, Mux8/1, Mux9/1, Mux10/1, Mux11/1, Mux12/1, Mux13/1
  Gsin/1 -> Mux2/2, Mux3/2, Mux4/2, Mux5/2, Mux6/2, Mux7/2, Mux8/2, Mux9/2, Mux10/2, Mux11/2, Mux12/2, Mux13/2
  Gsout/1 -> Mux2/3, Mux3/3, Mux4/3, Mux5/3, Mux6/3, Mux7/3, Mux8/3, Mux9/3, Mux10/3, Mux11/3, Mux12/3, Mux13/3
  rocm/1 -> Mux2/4, Mux3/4, Mux4/4, Mux5/4, Mux6/4, Mux7/4, Mux8/4, Mux9/4, Mux10/4, Mux11/4, Mux12/4, Mux13/4
  vol/1 -> Mux2/5, Mux3/5, Mux4/5, Mux5/5, Mux6/5, Mux7/5, Mux8/5, Mux9/5, Mux10/5, Mux11/5, Mux12/5, Mux13/5
  Mux3/1 -> MATLAB Fcn1/1
  MATLAB Fcn1/1 -> Integrator1/1
  Integrator1/1 -> Scope1/1, Mux3/7, Mux4/7, Mux5/7, Mux6/7, Mux7/7, Mux8/7, Mux9/7, Mux10/7, Mux11/7, Mux12/7, Mux13/7, Display1/1, Mux/3
  Mux4/1 -> MATLAB Fcn2/1
  MATLAB Fcn2/1 -> Integrator2/1
  Integrator2/1 -> Scope2/1, Mux4/8, Mux5/8, Mux6/8, Mux7/8, Mux8/8, Mux9/8, Mux10/8, Mux11/8, Mux12/8, Mux13/8, Display2/1, Mux/4
  MATLAB Fcn3/1 -> Integrator3/1
  Integrator3/1 -> Scope3/1, Mux5/9, Mux6/9, Mux7/9, Mux8/9, Mux9/9, Mux10/9, Mux11/9, Mux12/9, Mux13/9, Display3/1, Mux/5
  Mux5/1 -> MATLAB Fcn3/1
  Mux6/1 -> MATLAB Fcn4/1
  MATLAB Fcn4/1 -> Integrator4/1
  Integrator4/1 -> Scope4/1, Mux6/10, Mux7/10, Mux8/10, Mux9/10, Mux10/10, Mux11/10, Mux12/10, Mux13/10, Display4/1, Mux/6
  Mux7/1 -> MATLAB Fcn5/1
  MATLAB Fcn5/1 -> Integrator5/1
  Integrator5/1 -> Scope5/1, Mux7/11, Mux8/11, Mux9/11, Mux10/11, Mux11/11, Mux12/11, Mux13/11, Display5/1, Mux/7
  Mux8/1 -> MATLAB Fcn6/1
  MATLAB Fcn6/1 -> Integrator6/1
  Integrator6/1 -> Scope6/1, Mux8/12, Mux9/12, Mux10/12, Mux11/12, Mux12/12, Mux13/12, Display6/1, Mux/8
  Mux9/1 -> MATLAB Fcn7/1
  MATLAB Fcn7/1 -> Integrator7/1
  Integrator7/1 -> Scope7/1, Mux9/13, Mux10/13, Mux11/13, Mux12/13, Mux13/13, Display7/1, Mux/9
  Mux10/1 -> MATLAB Fcn8/1
  MATLAB Fcn8/1 -> Integrator8/1
  Integrator8/1 -> Scope8/1, Mux10/14, Mux11/14, Mux12/14, Mux13/14, Display8/1, Mux/10
  Mux11/1 -> MATLAB Fcn9/1
  MATLAB Fcn9/1 -> Integrator9/1
  Integrator9/1 -> Scope9/1, Mux11/15, Mux12/15, Mux13/15, Display9/1, Mux/11
  Mux12/1 -> MATLAB Fcn10/1
  MATLAB Fcn10/1 -> Integrator10/1
  Integrator10/1 -> Scope10/1, Mux12/16, Mux13/16, Display10/1, Mux/12
  Mux13/1 -> MATLAB Fcn11/1
  MATLAB Fcn11/1 -> Integrator11/1
  Integrator11/1 -> Scope11/1, Mux13/17, Display11/1, Mux/13
  Constant/1 -> Mux/1
  Mux/1 -> p3/1, Scope12/1
  P/1 -> Mux2/7, Mux3/8, Mux4/9, Mux5/10, Mux6/11, Mux7/12, Mux8/13, Mux9/14, Mux10/15, Mux11/16, Mux12/17, Mux13/18

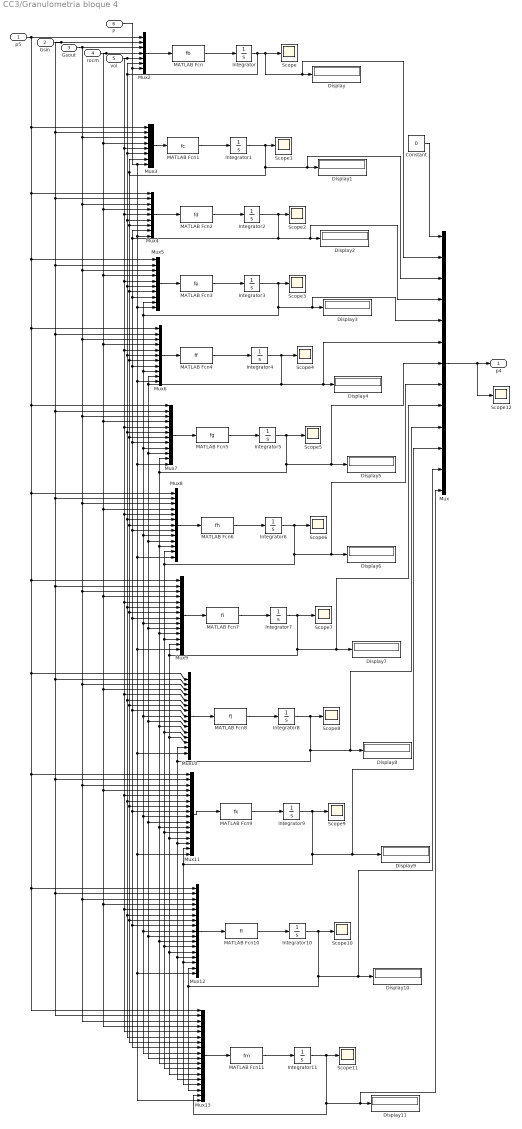
== system CC3/Granulometria bloque 4 ==
  p5 : Inport
  Gsin : Inport  Port=2
  Gsout : Inport  Port=3
  rocm : Inport  Port=4
  vol : Inport  Port=5
  P : Inport  Port=6
  Constant : Constant  Value=0  OutDataType=fixdt(1, 16)  OutScaling=2^0
  Display{,1..11} (12 alike) : Display
  Integrator{,1..11} (12 alike) : Integrator  InitialCondition=0.003
  MATLAB Fcn : MATLABFcn  MATLABFcn=fb
  MATLAB Fcn1 : MATLABFcn  MATLABFcn=fc
  MATLAB Fcn10 : MATLABFcn  MATLABFcn=fl
  MATLAB Fcn11 : MATLABFcn  MATLABFcn=fm
  MATLAB Fcn2 : MATLABFcn  MATLABFcn=fd
  MATLAB Fcn3 : MATLABFcn  MATLABFcn=fe
  MATLAB Fcn4 : MATLABFcn  MATLABFcn=ff
  MATLAB Fcn5 : MATLABFcn  MATLABFcn=fg
  MATLAB Fcn6 : MATLABFcn  MATLABFcn=fh
  MATLAB Fcn7 : MATLABFcn  MATLABFcn=fi
  MATLAB Fcn8 : MATLABFcn  MATLABFcn=fj
  MATLAB Fcn9 : MATLABFcn  MATLABFcn=fk
  Mux : Mux  Inputs=13
  Mux10 : Mux  Inputs=15
  Mux11 : Mux  Inputs=16
  Mux12 : Mux  Inputs=17
  Mux13 : Mux  Inputs=18
  Mux2 : Mux  Inputs=7
  Mux3 : Mux  Inputs=8
  Mux4 : Mux  Inputs=9
  Mux5 : Mux  Inputs=10
  Mux6 : Mux  Inputs=11
  Mux7 : Mux  Inputs=12
  Mux8 : Mux  Inputs=13
  Mux9 : Mux  Inputs=14
  Scope{,1..12} (13 alike) : Scope
      Scope settings: SaveName=ScopeData2
      Scope1 settings: SaveName=ScopeData20
      Scope10 settings: SaveName=ScopeData29
      Scope11 settings: SaveName=ScopeData30
      Scope12 settings: SaveName=ScopeData36
      Scope2 settings: SaveName=ScopeData21
      Scope3 settings: SaveName=ScopeData22
      Scope4 settings: SaveName=ScopeData23
      Scope5 settings: SaveName=ScopeData24
      Scope6 settings: SaveName=ScopeData25
      Scope7 settings: SaveName=ScopeData26
      Scope8 settings: SaveName=ScopeData27
      Scope9 settings: SaveName=ScopeData28
  p4 : Outport  OutDataType=fixdt(1, 16)  OutScaling=2^0
  wires:
  Mux2/1 -> MATLAB Fcn/1
  MATLAB Fcn/1 -> Integrator/1
  Integrator/1 -> Mux2/6, Mux3/6, Mux4/6, Mux5/6, Mux6/6, Mux7/6, Mux8/6, Mux9/6, Mux10/6, Mux11/6, Mux12/6, Mux13/6, Scope/1, Display/1, Mux/2
  p5/1 -> Mux2/1, Mux3/1, Mux4/1, Mux5/1, Mux6/1, Mux7/1, Mux8/1, Mux9/1, Mux10/1, Mux11/1, Mux12/1, Mux13/1
  Gsin/1 -> Mux2/2, Mux3/2, Mux4/2, Mux5/2, Mux6/2, Mux7/2, Mux8/2, Mux9/2, Mux10/2, Mux11/2, Mux12/2, Mux13/2
  Gsout/1 -> Mux2/3, Mux3/3, Mux4/3, Mux5/3, Mux6/3, Mux7/3, Mux8/3, Mux9/3, Mux10/3, Mux11/3, Mux12/3, Mux13/3
  rocm/1 -> Mux2/4, Mux3/4, Mux4/4, Mux5/4, Mux6/4, Mux7/4, Mux8/4, Mux9/4, Mux10/4, Mux11/4, Mux12/4, Mux13/4
  vol/1 -> Mux2/5, Mux3/5, Mux4/5, Mux5/5, Mux6/5, Mux7/5, Mux8/5, Mux9/5, Mux10/5, Mux11/5, Mux12/5, Mux13/5
  Mux3/1 -> MATLAB Fcn1/1
  MATLAB Fcn1/1 -> Integrator1/1
  Integrator1/1 -> Scope1/1, Mux3/7, Mux4/7, Mux5/7, Mux6/7, Mux7/7, Mux8/7, Mux9/7, Mux10/7, Mux11/7, Mux12/7, Mux13/7, Display1/1, Mux/3
  Mux4/1 -> MATLAB Fcn2/1
  MATLAB Fcn2/1 -> Integrator2/1
  Integrator2/1 -> Scope2/1, Mux4/8, Mux5/8, Mux6/8, Mux7/8, Mux8/8, Mux9/8, Mux10/8, Mux11/8, Mux12/8, Mux13/8, Display2/1, Mux/4
  MATLAB Fcn3/1 -> Integrator3/1
  Integrator3/1 -> Scope3/1, Mux5/9, Mux6/9, Mux7/9, Mux8/9, Mux9/9, Mux10/9, Mux11/9, Mux12/9, Mux13/9, Display3/1, Mux/5
  Mux5/1 -> MATLAB Fcn3/1
  Mux6/1 -> MATLAB Fcn4/1
  MATLAB Fcn4/1 -> Integrator4/1
  Integrator4/1 -> Scope4/1, Mux6/10, Mux7/10, Mux8/10, Mux9/10, Mux10/10, Mux11/10, Mux12/10, Mux13/10, Display4/1, Mux/6
  Mux7/1 -> MATLAB Fcn5/1
  MATLAB Fcn5/1 -> Integrator5/1
  Integrator5/1 -> Scope5/1, Mux7/11, Mux8/11, Mux9/11, Mux10/11, Mux11/11, Mux12/11, Mux13/11, Display5/1, Mux/7
  Mux8/1 -> MATLAB Fcn6/1
  MATLAB Fcn6/1 -> Integrator6/1
  Integrator6/1 -> Scope6/1, Mux8/12, Mux9/12, Mux10/12, Mux11/12, Mux12/12, Mux13/12, Display6/1, Mux/8
  Mux9/1 -> MATLAB Fcn7/1
  MATLAB Fcn7/1 -> Integrator7/1
  Integrator7/1 -> Scope7/1, Mux9/13, Mux10/13, Mux11/13, Mux12/13, Mux13/13, Display7/1, Mux/9
  Mux10/1 -> MATLAB Fcn8/1
  MATLAB Fcn8/1 -> Integrator8/1
  Integrator8/1 -> Scope8/1, Mux10/14, Mux11/14, Mux12/14, Mux13/14, Display8/1, Mux/10
  Mux11/1 -> MATLAB Fcn9/1
  MATLAB Fcn9/1 -> Integrator9/1
  Integrator9/1 -> Scope9/1, Mux11/15, Mux12/15, Mux13/15, Display9/1, Mux/11
  Mux12/1 -> MATLAB Fcn10/1
  MATLAB Fcn10/1 -> Integrator10/1
  Integrator10/1 -> Scope10/1, Mux12/16, Mux13/16, Display10/1, Mux/12
  Mux13/1 -> MATLAB Fcn11/1
  MATLAB Fcn11/1 -> Integrator11/1
  Integrator11/1 -> Scope11/1, Mux13/17, Display11/1, Mux/13
  Constant/1 -> Mux/1
  Mux/1 -> p4/1, Scope12/1
  P/1 -> Mux2/7, Mux3/8, Mux4/9, Mux5/10, Mux6/11, Mux7/12, Mux8/13, Mux9/14, Mux10/15, Mux11/16, Mux12/17, Mux13/18

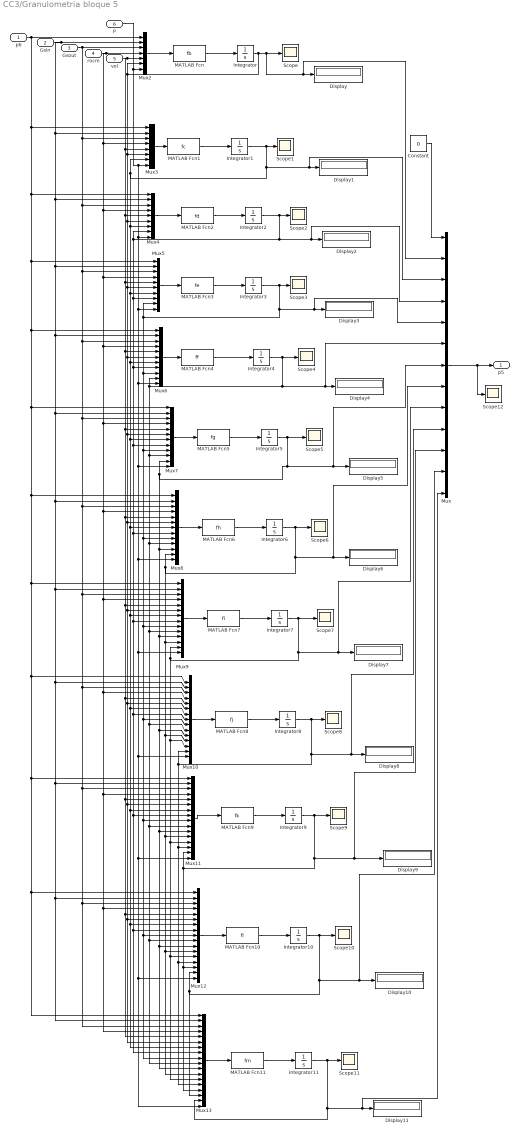
== system CC3/Granulometria bloque 5 ==
  p6 : Inport
  Gsin : Inport  Port=2
  Gsout : Inport  Port=3
  rocm : Inport  Port=4
  vol : Inport  Port=5
  P : Inport  Port=6
  Constant : Constant  Value=0  OutDataType=fixdt(1, 16)  OutScaling=2^0
  Display{,1..11} (12 alike) : Display
  Integrator{,1..11} (12 alike) : Integrator  InitialCondition=0.003
  MATLAB Fcn : MATLABFcn  MATLABFcn=fb
  MATLAB Fcn1 : MATLABFcn  MATLABFcn=fc
  MATLAB Fcn10 : MATLABFcn  MATLABFcn=fl
  MATLAB Fcn11 : MATLABFcn  MATLABFcn=fm
  MATLAB Fcn2 : MATLABFcn  MATLABFcn=fd
  MATLAB Fcn3 : MATLABFcn  MATLABFcn=fe
  MATLAB Fcn4 : MATLABFcn  MATLABFcn=ff
  MATLAB Fcn5 : MATLABFcn  MATLABFcn=fg
  MATLAB Fcn6 : MATLABFcn  MATLABFcn=fh
  MATLAB Fcn7 : MATLABFcn  MATLABFcn=fi
  MATLAB Fcn8 : MATLABFcn  MATLABFcn=fj
  MATLAB Fcn9 : MATLABFcn  MATLABFcn=fk
  Mux : Mux  Inputs=13
  Mux10 : Mux  Inputs=15
  Mux11 : Mux  Inputs=16
  Mux12 : Mux  Inputs=17
  Mux13 : Mux  Inputs=18
  Mux2 : Mux  Inputs=7
  Mux3 : Mux  Inputs=8
  Mux4 : Mux  Inputs=9
  Mux5 : Mux  Inputs=10
  Mux6 : Mux  Inputs=11
  Mux7 : Mux  Inputs=12
  Mux8 : Mux  Inputs=13
  Mux9 : Mux  Inputs=14
  Scope{,1..12} (13 alike) : Scope
      Scope settings: SaveName=ScopeData2
      Scope1 settings: SaveName=ScopeData20
      Scope10 settings: SaveName=ScopeData29
      Scope11 settings: SaveName=ScopeData30
      Scope12 settings: SaveName=ScopeData35
      Scope2 settings: SaveName=ScopeData21
      Scope3 settings: SaveName=ScopeData22
      Scope4 settings: SaveName=ScopeData23
      Scope5 settings: SaveName=ScopeData24
      Scope6 settings: SaveName=ScopeData25
      Scope7 settings: SaveName=ScopeData26
      Scope8 settings: SaveName=ScopeData27
      Scope9 settings: SaveName=ScopeData28
  p5 : Outport  OutDataType=fixdt(1, 16)  OutScaling=2^0
  wires:
  Mux2/1 -> MATLAB Fcn/1
  MATLAB Fcn/1 -> Integrator/1
  Integrator/1 -> Mux2/6, Mux3/6, Mux4/6, Mux5/6, Mux6/6, Mux7/6, Mux8/6, Mux9/6, Mux10/6, Mux11/6, Mux12/6, Mux13/6, Scope/1, Display/1, Mux/2
  p6/1 -> Mux2/1, Mux3/1, Mux4/1, Mux5/1, Mux6/1, Mux7/1, Mux8/1, Mux9/1, Mux10/1, Mux11/1, Mux12/1, Mux13/1
  Gsin/1 -> Mux2/2, Mux3/2, Mux4/2, Mux5/2, Mux6/2, Mux7/2, Mux8/2, Mux9/2, Mux10/2, Mux11/2, Mux12/2, Mux13/2
  Gsout/1 -> Mux2/3, Mux3/3, Mux4/3, Mux5/3, Mux6/3, Mux7/3, Mux8/3, Mux9/3, Mux10/3, Mux11/3, Mux12/3, Mux13/3
  rocm/1 -> Mux2/4, Mux3/4, Mux4/4, Mux5/4, Mux6/4, Mux7/4, Mux8/4, Mux9/4, Mux10/4, Mux11/4, Mux12/4, Mux13/4
  vol/1 -> Mux2/5, Mux3/5, Mux4/5, Mux5/5, Mux6/5, Mux7/5, Mux8/5, Mux9/5, Mux10/5, Mux11/5, Mux12/5, Mux13/5
  Mux3/1 -> MATLAB Fcn1/1
  MATLAB Fcn1/1 -> Integrator1/1
  Integrator1/1 -> Scope1/1, Mux3/7, Mux4/7, Mux5/7, Mux6/7, Mux7/7, Mux8/7, Mux9/7, Mux10/7, Mux11/7, Mux12/7, Mux13/7, Display1/1, Mux/3
  Mux4/1 -> MATLAB Fcn2/1
  MATLAB Fcn2/1 -> Integrator2/1
  Integrator2/1 -> Scope2/1, Mux4/8, Mux5/8, Mux6/8, Mux7/8, Mux8/8, Mux9/8, Mux10/8, Mux11/8, Mux12/8, Mux13/8, Display2/1, Mux/4
  MATLAB Fcn3/1 -> Integrator3/1
  Integrator3/1 -> Scope3/1, Mux5/9, Mux6/9, Mux7/9, Mux8/9, Mux9/9, Mux10/9, Mux11/9, Mux12/9, Mux13/9, Display3/1, Mux/5
  Mux5/1 -> MATLAB Fcn3/1
  Mux6/1 -> MATLAB Fcn4/1
  MATLAB Fcn4/1 -> Integrator4/1
  Integrator4/1 -> Scope4/1, Mux6/10, Mux7/10, Mux8/10, Mux9/10, Mux10/10, Mux11/10, Mux12/10, Mux13/10, Display4/1, Mux/6
  Mux7/1 -> MATLAB Fcn5/1
  MATLAB Fcn5/1 -> Integrator5/1
  Integrator5/1 -> Scope5/1, Mux7/11, Mux8/11, Mux9/11, Mux10/11, Mux11/11, Mux12/11, Mux13/11, Display5/1, Mux/7
  Mux8/1 -> MATLAB Fcn6/1
  MATLAB Fcn6/1 -> Integrator6/1
  Integrator6/1 -> Scope6/1, Mux8/12, Mux9/12, Mux10/12, Mux11/12, Mux12/12, Mux13/12, Display6/1, Mux/8
  Mux9/1 -> MATLAB Fcn7/1
  MATLAB Fcn7/1 -> Integrator7/1
  Integrator7/1 -> Scope7/1, Mux9/13, Mux10/13, Mux11/13, Mux12/13, Mux13/13, Display7/1, Mux/9
  Mux10/1 -> MATLAB Fcn8/1
  MATLAB Fcn8/1 -> Integrator8/1
  Integrator8/1 -> Scope8/1, Mux10/14, Mux11/14, Mux12/14, Mux13/14, Display8/1, Mux/10
  Mux11/1 -> MATLAB Fcn9/1
  MATLAB Fcn9/1 -> Integrator9/1
  Integrator9/1 -> Scope9/1, Mux11/15, Mux12/15, Mux13/15, Display9/1, Mux/11
  Mux12/1 -> MATLAB Fcn10/1
  MATLAB Fcn10/1 -> Integrator10/1
  Integrator10/1 -> Scope10/1, Mux12/16, Mux13/16, Display10/1, Mux/12
  Mux13/1 -> MATLAB Fcn11/1
  MATLAB Fcn11/1 -> Integrator11/1
  Integrator11/1 -> Scope11/1, Mux13/17, Display11/1, Mux/13
  Constant/1 -> Mux/1
  Mux/1 -> p5/1, Scope12/1
  P/1 -> Mux2/7, Mux3/8, Mux4/9, Mux5/10, Mux6/11, Mux7/12, Mux8/13, Mux9/14, Mux10/15, Mux11/16, Mux12/17, Mux13/18

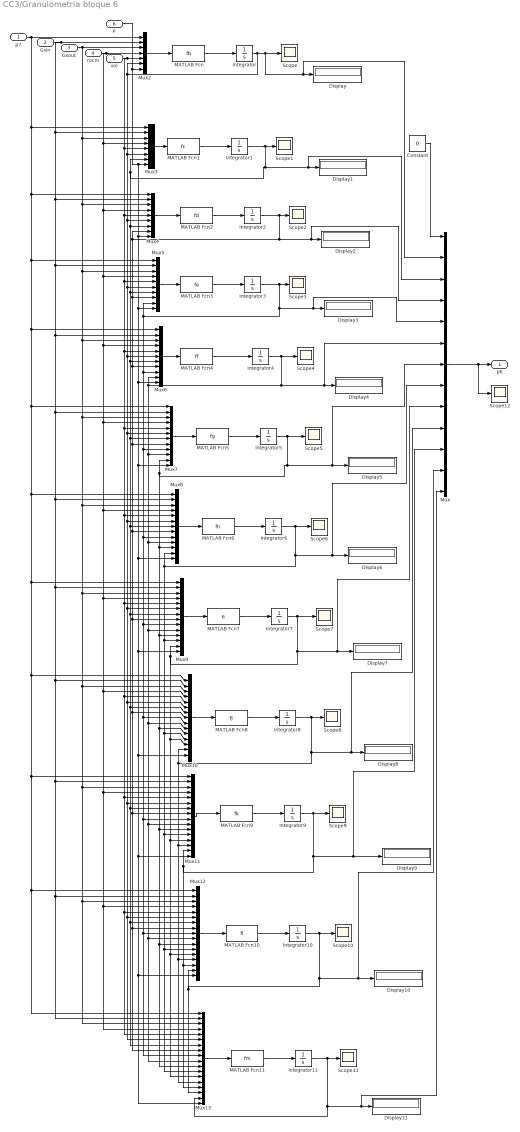
== system CC3/Granulometria bloque 6 ==
  p7 : Inport
  Gsin : Inport  Port=2
  Gsout : Inport  Port=3
  rocm : Inport  Port=4
  vol : Inport  Port=5
  P : Inport  Port=6
  Constant : Constant  Value=0  OutDataType=fixdt(1, 16)  OutScaling=2^0
  Display{,1..11} (12 alike) : Display
  Integrator{,1..11} (12 alike) : Integrator  InitialCondition=0.003
  MATLAB Fcn : MATLABFcn  MATLABFcn=fb
  MATLAB Fcn1 : MATLABFcn  MATLABFcn=fc
  MATLAB Fcn10 : MATLABFcn  MATLABFcn=fl
  MATLAB Fcn11 : MATLABFcn  MATLABFcn=fm
  MATLAB Fcn2 : MATLABFcn  MATLABFcn=fd
  MATLAB Fcn3 : MATLABFcn  MATLABFcn=fe
  MATLAB Fcn4 : MATLABFcn  MATLABFcn=ff
  MATLAB Fcn5 : MATLABFcn  MATLABFcn=fg
  MATLAB Fcn6 : MATLABFcn  MATLABFcn=fh
  MATLAB Fcn7 : MATLABFcn  MATLABFcn=fi
  MATLAB Fcn8 : MATLABFcn  MATLABFcn=fj
  MATLAB Fcn9 : MATLABFcn  MATLABFcn=fk
  Mux : Mux  Inputs=13
  Mux10 : Mux  Inputs=15
  Mux11 : Mux  Inputs=16
  Mux12 : Mux  Inputs=17
  Mux13 : Mux  Inputs=18
  Mux2 : Mux  Inputs=7
  Mux3 : Mux  Inputs=8
  Mux4 : Mux  Inputs=9
  Mux5 : Mux  Inputs=10
  Mux6 : Mux  Inputs=11
  Mux7 : Mux  Inputs=12
  Mux8 : Mux  Inputs=13
  Mux9 : Mux  Inputs=14
  Scope{,1..12} (13 alike) : Scope
      Scope settings: SaveName=ScopeData2
      Scope1 settings: SaveName=ScopeData20
      Scope10 settings: SaveName=ScopeData29
      Scope11 settings: SaveName=ScopeData30
      Scope12 settings: SaveName=ScopeData34
      Scope2 settings: SaveName=ScopeData21
      Scope3 settings: SaveName=ScopeData22
      Scope4 settings: SaveName=ScopeData23
      Scope5 settings: SaveName=ScopeData24
      Scope6 settings: SaveName=ScopeData25
      Scope7 settings: SaveName=ScopeData26
      Scope8 settings: SaveName=ScopeData27
      Scope9 settings: SaveName=ScopeData28
  p6 : Outport  OutDataType=fixdt(1, 16)  OutScaling=2^0
  wires:
  Mux2/1 -> MATLAB Fcn/1
  MATLAB Fcn/1 -> Integrator/1
  Integrator/1 -> Mux2/6, Mux3/6, Mux4/6, Mux5/6, Mux6/6, Mux7/6, Mux8/6, Mux9/6, Mux10/6, Mux11/6, Mux12/6, Mux13/6, Scope/1, Display/1, Mux/2
  p7/1 -> Mux2/1, Mux3/1, Mux4/1, Mux5/1, Mux6/1, Mux7/1, Mux8/1, Mux9/1, Mux10/1, Mux11/1, Mux12/1, Mux13/1
  Gsin/1 -> Mux2/2, Mux3/2, Mux4/2, Mux5/2, Mux6/2, Mux7/2, Mux8/2, Mux9/2, Mux10/2, Mux11/2, Mux12/2, Mux13/2
  Gsout/1 -> Mux2/3, Mux3/3, Mux4/3, Mux5/3, Mux6/3, Mux7/3, Mux8/3, Mux9/3, Mux10/3, Mux11/3, Mux12/3, Mux13/3
  rocm/1 -> Mux2/4, Mux3/4, Mux4/4, Mux5/4, Mux6/4, Mux7/4, Mux8/4, Mux9/4, Mux10/4, Mux11/4, Mux12/4, Mux13/4
  vol/1 -> Mux2/5, Mux3/5, Mux4/5, Mux5/5, Mux6/5, Mux7/5, Mux8/5, Mux9/5, Mux10/5, Mux11/5, Mux12/5, Mux13/5
  Mux3/1 -> MATLAB Fcn1/1
  MATLAB Fcn1/1 -> Integrator1/1
  Integrator1/1 -> Scope1/1, Mux3/7, Mux4/7, Mux5/7, Mux6/7, Mux7/7, Mux8/7, Mux9/7, Mux10/7, Mux11/7, Mux12/7, Mux13/7, Display1/1, Mux/3
  Mux4/1 -> MATLAB Fcn2/1
  MATLAB Fcn2/1 -> Integrator2/1
  Integrator2/1 -> Scope2/1, Mux4/8, Mux5/8, Mux6/8, Mux7/8, Mux8/8, Mux9/8, Mux10/8, Mux11/8, Mux12/8, Mux13/8, Display2/1, Mux/4
  MATLAB Fcn3/1 -> Integrator3/1
  Integrator3/1 -> Scope3/1, Mux5/9, Mux6/9, Mux7/9, Mux8/9, Mux9/9, Mux10/9, Mux11/9, Mux12/9, Mux13/9, Display3/1, Mux/5
  Mux5/1 -> MATLAB Fcn3/1
  Mux6/1 -> MATLAB Fcn4/1
  MATLAB Fcn4/1 -> Integrator4/1
  Integrator4/1 -> Scope4/1, Mux6/10, Mux7/10, Mux8/10, Mux9/10, Mux10/10, Mux11/10, Mux12/10, Mux13/10, Display4/1, Mux/6
  Mux7/1 -> MATLAB Fcn5/1
  MATLAB Fcn5/1 -> Integrator5/1
  Integrator5/1 -> Scope5/1, Mux7/11, Mux8/11, Mux9/11, Mux10/11, Mux11/11, Mux12/11, Mux13/11, Display5/1, Mux/7
  Mux8/1 -> MATLAB Fcn6/1
  MATLAB Fcn6/1 -> Integrator6/1
  Integrator6/1 -> Scope6/1, Mux8/12, Mux9/12, Mux10/12, Mux11/12, Mux12/12, Mux13/12, Display6/1, Mux/8
  Mux9/1 -> MATLAB Fcn7/1
  MATLAB Fcn7/1 -> Integrator7/1
  Integrator7/1 -> Scope7/1, Mux9/13, Mux10/13, Mux11/13, Mux12/13, Mux13/13, Display7/1, Mux/9
  Mux10/1 -> MATLAB Fcn8/1
  MATLAB Fcn8/1 -> Integrator8/1
  Integrator8/1 -> Scope8/1, Mux10/14, Mux11/14, Mux12/14, Mux13/14, Display8/1, Mux/10
  Mux11/1 -> MATLAB Fcn9/1
  MATLAB Fcn9/1 -> Integrator9/1
  Integrator9/1 -> Scope9/1, Mux11/15, Mux12/15, Mux13/15, Display9/1, Mux/11
  Mux12/1 -> MATLAB Fcn10/1
  MATLAB Fcn10/1 -> Integrator10/1
  Integrator10/1 -> Scope10/1, Mux12/16, Mux13/16, Display10/1, Mux/12
  Mux13/1 -> MATLAB Fcn11/1
  MATLAB Fcn11/1 -> Integrator11/1
  Integrator11/1 -> Scope11/1, Mux13/17, Display11/1, Mux/13
  Constant/1 -> Mux/1
  Mux/1 -> p6/1, Scope12/1
  P/1 -> Mux2/7, Mux3/8, Mux4/9, Mux5/10, Mux6/11, Mux7/12, Mux8/13, Mux9/14, Mux10/15, Mux11/16, Mux12/17, Mux13/18

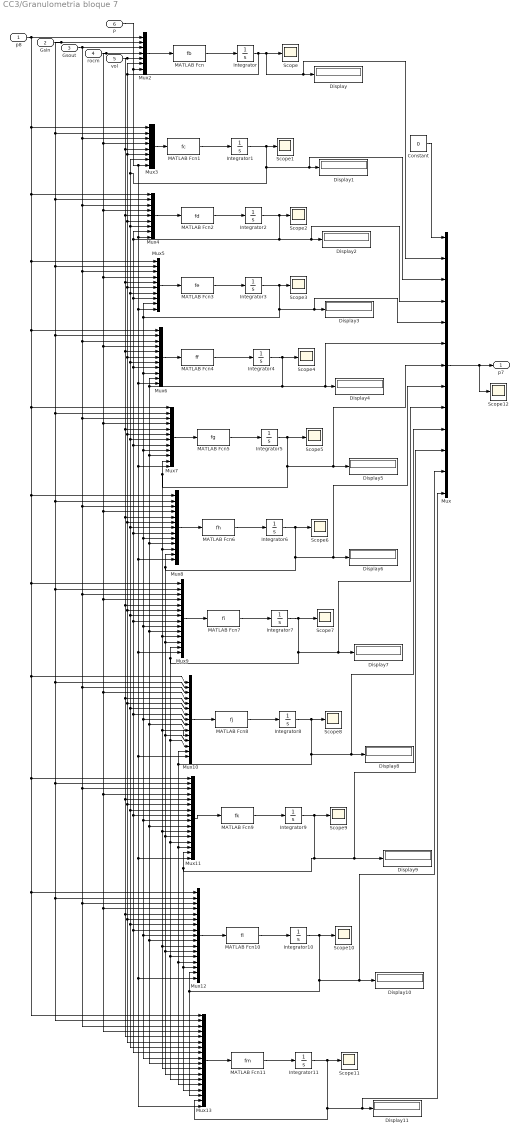
== system CC3/Granulometria bloque 7 ==
  p8 : Inport
  Gsin : Inport  Port=2
  Gsout : Inport  Port=3
  rocm : Inport  Port=4
  vol : Inport  Port=5
  P : Inport  Port=6
  Constant : Constant  Value=0  OutDataType=fixdt(1, 16)  OutScaling=2^0
  Display{,1..11} (12 alike) : Display
  Integrator{,1..11} (12 alike) : Integrator  InitialCondition=0.003
  MATLAB Fcn : MATLABFcn  MATLABFcn=fb
  MATLAB Fcn1 : MATLABFcn  MATLABFcn=fc
  MATLAB Fcn10 : MATLABFcn  MATLABFcn=fl
  MATLAB Fcn11 : MATLABFcn  MATLABFcn=fm
  MATLAB Fcn2 : MATLABFcn  MATLABFcn=fd
  MATLAB Fcn3 : MATLABFcn  MATLABFcn=fe
  MATLAB Fcn4 : MATLABFcn  MATLABFcn=ff
  MATLAB Fcn5 : MATLABFcn  MATLABFcn=fg
  MATLAB Fcn6 : MATLABFcn  MATLABFcn=fh
  MATLAB Fcn7 : MATLABFcn  MATLABFcn=fi
  MATLAB Fcn8 : MATLABFcn  MATLABFcn=fj
  MATLAB Fcn9 : MATLABFcn  MATLABFcn=fk
  Mux : Mux  Inputs=13
  Mux10 : Mux  Inputs=15
  Mux11 : Mux  Inputs=16
  Mux12 : Mux  Inputs=17
  Mux13 : Mux  Inputs=18
  Mux2 : Mux  Inputs=7
  Mux3 : Mux  Inputs=8
  Mux4 : Mux  Inputs=9
  Mux5 : Mux  Inputs=10
  Mux6 : Mux  Inputs=11
  Mux7 : Mux  Inputs=12
  Mux8 : Mux  Inputs=13
  Mux9 : Mux  Inputs=14
  Scope{,1..12} (13 alike) : Scope
      Scope settings: SaveName=ScopeData2
      Scope1 settings: SaveName=ScopeData20
      Scope10 settings: SaveName=ScopeData29
      Scope11 settings: SaveName=ScopeData30
      Scope12 settings: SaveName=ScopeData33
      Scope2 settings: SaveName=ScopeData21
      Scope3 settings: SaveName=ScopeData22
      Scope4 settings: SaveName=ScopeData23
      Scope5 settings: SaveName=ScopeData24
      Scope6 settings: SaveName=ScopeData25
      Scope7 settings: SaveName=ScopeData26
      Scope8 settings: SaveName=ScopeData27
      Scope9 settings: SaveName=ScopeData28
  p7 : Outport  OutDataType=fixdt(1, 16)  OutScaling=2^0
  wires:
  Mux2/1 -> MATLAB Fcn/1
  MATLAB Fcn/1 -> Integrator/1
  Integrator/1 -> Mux2/6, Mux3/6, Mux4/6, Mux5/6, Mux6/6, Mux7/6, Mux8/6, Mux9/6, Mux10/6, Mux11/6, Mux12/6, Mux13/6, Scope/1, Display/1, Mux/2
  p8/1 -> Mux2/1, Mux3/1, Mux4/1, Mux5/1, Mux6/1, Mux7/1, Mux8/1, Mux9/1, Mux10/1, Mux11/1, Mux12/1, Mux13/1
  Gsin/1 -> Mux2/2, Mux3/2, Mux4/2, Mux5/2, Mux6/2, Mux7/2, Mux8/2, Mux9/2, Mux10/2, Mux11/2, Mux12/2, Mux13/2
  Gsout/1 -> Mux2/3, Mux3/3, Mux4/3, Mux5/3, Mux6/3, Mux7/3, Mux8/3, Mux9/3, Mux10/3, Mux11/3, Mux12/3, Mux13/3
  rocm/1 -> Mux2/4, Mux3/4, Mux4/4, Mux5/4, Mux6/4, Mux7/4, Mux8/4, Mux9/4, Mux10/4, Mux11/4, Mux12/4, Mux13/4
  vol/1 -> Mux2/5, Mux3/5, Mux4/5, Mux5/5, Mux6/5, Mux7/5, Mux8/5, Mux9/5, Mux10/5, Mux11/5, Mux12/5, Mux13/5
  Mux3/1 -> MATLAB Fcn1/1
  MATLAB Fcn1/1 -> Integrator1/1
  Integrator1/1 -> Scope1/1, Mux3/7, Mux4/7, Mux5/7, Mux6/7, Mux7/7, Mux8/7, Mux9/7, Mux10/7, Mux11/7, Mux12/7, Mux13/7, Display1/1, Mux/3
  Mux4/1 -> MATLAB Fcn2/1
  MATLAB Fcn2/1 -> Integrator2/1
  Integrator2/1 -> Scope2/1, Mux4/8, Mux5/8, Mux6/8, Mux7/8, Mux8/8, Mux9/8, Mux10/8, Mux11/8, Mux12/8, Mux13/8, Display2/1, Mux/4
  MATLAB Fcn3/1 -> Integrator3/1
  Integrator3/1 -> Scope3/1, Mux5/9, Mux6/9, Mux7/9, Mux8/9, Mux9/9, Mux10/9, Mux11/9, Mux12/9, Mux13/9, Display3/1, Mux/5
  Mux5/1 -> MATLAB Fcn3/1
  Mux6/1 -> MATLAB Fcn4/1
  MATLAB Fcn4/1 -> Integrator4/1
  Integrator4/1 -> Scope4/1, Mux6/10, Mux7/10, Mux8/10, Mux9/10, Mux10/10, Mux11/10, Mux12/10, Mux13/10, Display4/1, Mux/6
  Mux7/1 -> MATLAB Fcn5/1
  MATLAB Fcn5/1 -> Integrator5/1
  Integrator5/1 -> Scope5/1, Mux7/11, Mux8/11, Mux9/11, Mux10/11, Mux11/11, Mux12/11, Mux13/11, Display5/1, Mux/7
  Mux8/1 -> MATLAB Fcn6/1
  MATLAB Fcn6/1 -> Integrator6/1
  Integrator6/1 -> Scope6/1, Mux8/12, Mux9/12, Mux10/12, Mux11/12, Mux12/12, Mux13/12, Display6/1, Mux/8
  Mux9/1 -> MATLAB Fcn7/1
  MATLAB Fcn7/1 -> Integrator7/1
  Integrator7/1 -> Scope7/1, Mux9/13, Mux10/13, Mux11/13, Mux12/13, Mux13/13, Display7/1, Mux/9
  Mux10/1 -> MATLAB Fcn8/1
  MATLAB Fcn8/1 -> Integrator8/1
  Integrator8/1 -> Scope8/1, Mux10/14, Mux11/14, Mux12/14, Mux13/14, Display8/1, Mux/10
  Mux11/1 -> MATLAB Fcn9/1
  MATLAB Fcn9/1 -> Integrator9/1
  Integrator9/1 -> Scope9/1, Mux11/15, Mux12/15, Mux13/15, Display9/1, Mux/11
  Mux12/1 -> MATLAB Fcn10/1
  MATLAB Fcn10/1 -> Integrator10/1
  Integrator10/1 -> Scope10/1, Mux12/16, Mux13/16, Display10/1, Mux/12
  Mux13/1 -> MATLAB Fcn11/1
  MATLAB Fcn11/1 -> Integrator11/1
  Integrator11/1 -> Scope11/1, Mux13/17, Display11/1, Mux/13
  Constant/1 -> Mux/1
  Mux/1 -> p7/1, Scope12/1
  P/1 -> Mux2/7, Mux3/8, Mux4/9, Mux5/10, Mux6/11, Mux7/12, Mux8/13, Mux9/14, Mux10/15, Mux11/16, Mux12/17, Mux13/18
